simulink model "schema_sistema_regolato"  (Simulink 7.6)
settings: Solver=ode45  StartTime=0.0  StopTime=10.0  MaxStep=0.01  RelTol=1e-3
values from neighbouring files (symbols this model uses):
  A = [0 1;-k/M -h/M]    [es1_ctrl_obs_massa.m]    (also in es2_ctrl_obs_altro.m = [2 3;4 1])
  B = [0;1/M]    [es1_ctrl_obs_massa.m]    (also in es2_ctrl_obs_altro.m = [1;0])
  C = [1 0]    [es1_ctrl_obs_massa.m]    (also in es2_ctrl_obs_altro.m)
  D = 0    [es1_ctrl_obs_massa.m]    (also in es2_ctrl_obs_altro.m)
  K = -place(A,B,aval_des)    [es1_ctrl_obs_massa.m]    (also in es2_ctrl_obs_altro.m = [k1 k2])
  ueq = 3    [es1_ctrl_obs_massa.m]    (also in es2_ctrl_obs_altro.m = 1)
  x0 = [1;0]    [es1_ctrl_obs_massa.m]    (also in es2_ctrl_obs_altro.m = [1;1])
  xeq = [0;0]    [es1_ctrl_obs_massa.m]    (also in es2_ctrl_obs_altro.m)
libraries: simulink x1
settings Model: Creator=professore  LastModifiedBy=patrizio

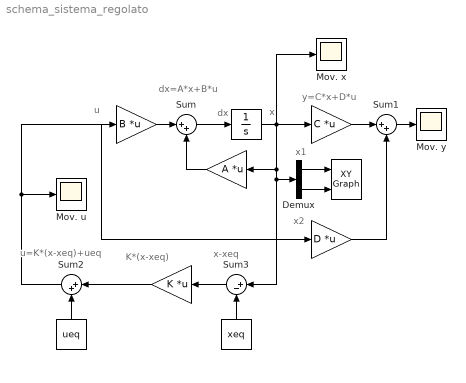
== system schema_sistema_regolato ==
  note: dx=A*x+B*u
  note: y=C*x+D*u
  note: u=K*(x-xeq)+ueq
  note: dx
  note: x
  note: u
  note: K*(x-xeq)
  note: x-xeq
  note: x1
  note: x2
  " " : Constant  Value=ueq
  "  " : Gain  Gain=K  Multiplication=Matrix(K*u)
  "   " : Constant  Value=xeq
  "     " : Gain  Gain=D  Multiplication=Matrix(K*u)
  "       " : simulink/Sinks/XY Graph  SystemSampleTime=-1  xmin=1  xmax=1.5  ymin=0  ymax=2  st=-1
  "        " : Gain  Gain=A  Multiplication=Matrix(K*u)
  "         " : Gain  Gain=B  Multiplication=Matrix(K*u)
  "          " : Gain  Gain=C  Multiplication=Matrix(K*u)
  "           " : Integrator  InitialCondition=x0
  Demux : Demux  Outputs=2
  Mov. u : Scope
      settings: SaveName=ScopeData2
  Mov. x : Scope
  Mov. y : Scope
  Sum : Sum  Inputs=|++
  Sum1 : Sum  Inputs=|++
  Sum2 : Sum  Inputs=|++
  Sum3 : Sum  Inputs=|+-
  wires:
  "         "/1 -> Sum/1
  "        "/1 -> Sum/2
  Sum/1 -> "           "/1
  "           "/1 -> "          "/1, "        "/1, Sum3/1, Demux/1, Mov. x/1
  "          "/1 -> Sum1/1
  "     "/1 -> Sum1/2
  "  "/1 -> Sum2/1
  " "/1 -> Sum2/2
  Sum3/1 -> "  "/1
  "   "/1 -> Sum3/2
  Sum2/1 -> "         "/1, "     "/1, Mov. u/1
  Sum1/1 -> Mov. y/1
  Demux/1 -> "       "/1
  Demux/2 -> "       "/2
